simulink model "Problem4"  (R2020a)
settings: Solver=VariableStepAuto  StartTime=0.0  StopTime=10.0  RelTol=1e-3
settings Model: Creator=Shreyas  LastModifiedBy=Shreyas

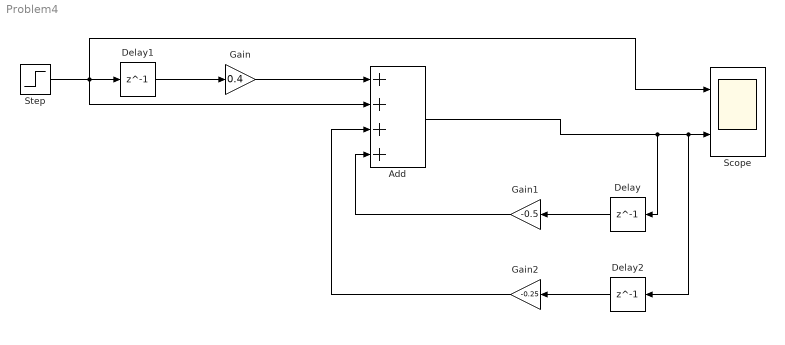
== system Problem4 ==
  Add : Sum  Inputs=++++
  Delay : Delay  DelayLength=1
  Delay1 : Delay  DelayLength=1
  Delay2 : Delay  DelayLength=1
  Gain : Gain  Gain=0.4
  Gain1 : Gain  Gain=-0.5
  Gain2 : Gain  Gain=-0.25
  Scope : Scope  NumInputPorts=2
  Step : Step  SampleTime=0
  wires:
  Delay1/1 -> Gain/1
  Step/1 -> Add/2, Scope/1, Delay1/1
  Gain/1 -> Add/1
  Add/1 -> Delay/1, Delay2/1, Scope/2
  Delay/1 -> Gain1/1
  Delay2/1 -> Gain2/1
  Gain1/1 -> Add/4
  Gain2/1 -> Add/3
